simulink model "plant"  (R2021b)
settings: Solver=VariableStepAuto  StartTime=0.0  StopTime=10.0  RelTol=1e-3
settings Model: Creator=DAUIN-Win10  LastModifiedBy=maria

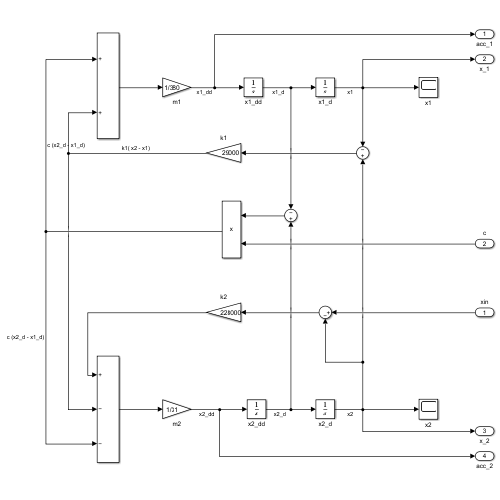
[thumbnail: Simulink's stored preview of the top-level diagram]
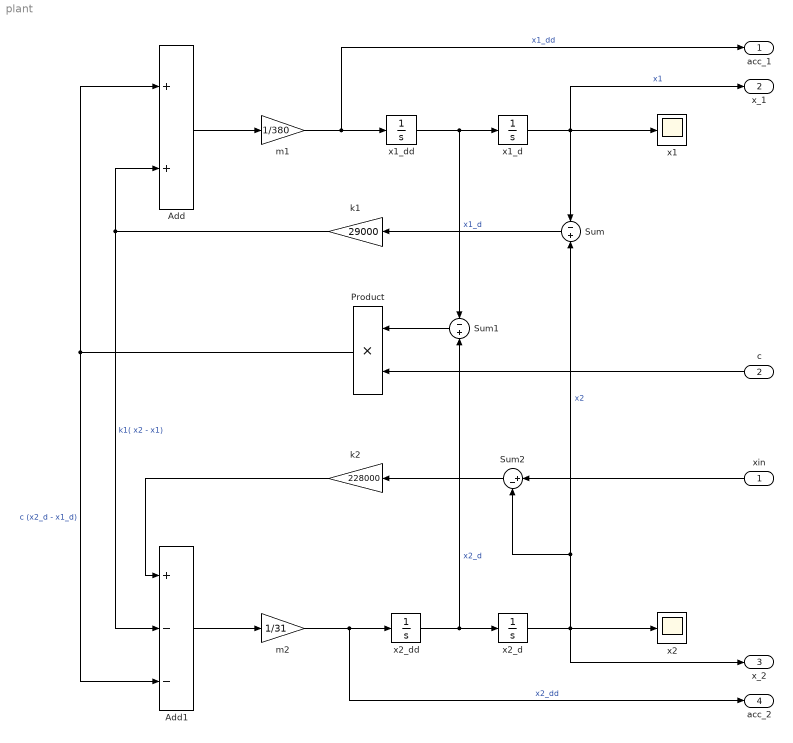
== system plant ==
  xin : Inport  OutMin=-0.2  OutMax=0.2  OutDataTypeStr=double
  c : Inport  Port=2  OutDataTypeStr=boolean
  Add : Sum
  Add1 : Sum  Inputs=+--
  Product : Product
  Sum : Sum  Inputs=-+
  Sum1 : Sum  Inputs=-+
  Sum2 : Sum  Inputs=|+-
  k1 : Gain  Gain=29000
  k2 : Gain  Gain=228000
  m1 : Gain  Gain=1/380
  m2 : Gain  Gain=1/31
  x1 : Scope
  x1_d : Integrator
  x1_dd : Integrator
  x2 : Scope
  x2_d : Integrator
  x2_dd : Integrator
  acc_1 : Outport  OutDataTypeStr=double
  x_1 : Outport  Port=2  OutDataTypeStr=double
  x_2 : Outport  Port=3  OutDataTypeStr=double
  acc_2 : Outport  Port=4  OutDataTypeStr=double
  wires:
  Add/1 -> m1/1
  x1_dd/1 -> Sum1/1, x1_d/1  "x1_d"
  xin/1 -> Sum2/1
  Add1/1 -> m2/1
  Sum/1 -> k1/1
  x2_dd/1 -> x2_d/1, Sum1/2  "x2_d"
  x1_d/1 -> x1/1, Sum/1, x_1/1  "x1"
  m1/1 -> acc_1/1, x1_dd/1  "x1_dd"
  k2/1 -> Add1/1
  x2_d/1 -> x2/1, x_2/1, Sum2/2, Sum/2  "x2"
  k1/1 -> Add1/2, Add/2  "k1( x2 - x1)"
  m2/1 -> acc_2/1, x2_dd/1  "x2_dd"
  Product/1 -> Add1/3, Add/1  "c (x2_d - x1_d)"
  c/1 -> Product/2
  Sum2/1 -> k2/1
  Sum1/1 -> Product/1
